simulink model "SimNL_Subsystems"  (R2016b)
settings: Solver=VariableStepAuto  StartTime=0.0  StopTime=10  FixedStep=SampleTime  RelTol=1e-3
values from neighbouring files (symbols this model uses):
  AC = []    [SetupNL.m]
undefined symbols (not defined in the file or in its folder): Env, Sim
libraries: OpenFlightUtilLib x17, SimCoreLib x3
(part 1 of 2)
settings Model: LastModifiedBy=rega0051
settings SolverCC: AlgebraicLoopSolver=LineSearch  AutoInsertRateTranBlk=on
settings DataIOCC: ExternalInput=simIn  FinalStateName=simStatesFinal  InitialState=simStatesInit  SaveOutput=off  SignalLogging=off  DSMLogging=off  StreamVariableName=simStream  SaveTime=off  StateSaveName=simStates  TimeSaveName=simTime  OutputSaveName=simOut  SignalLoggingName=simLog  DSMLoggingName=simData
settings OptimizationCC: ExpressionDepthLimit=2147483647  LifeSpan=inf
settings DebuggingCC: SignalInfNanChecking=warning  SaveWithParameterizedLinksMsg=none  UnderspecifiedInitializationDetection=Classic  MergeDetectMultiDrivingBlocksExec=none  CheckMatrixSingularityMsg=warning  UnnecessaryDatatypeConvMsg=warning  SignalLabelMismatchMsg=warning  SFcnCompatibilityMsg=warning  UniqueDataStoreMsg=error  ModelReferenceIOMsg=warning  ModelReferenceVersionMismatchMessage=warning  ModelReferenceIOMismatchMessage=warning  ModelReferenceExtraNoncontSigs=none  StateNameClashWarn=warning  StrictBusMsg=WarnOnBusTreatedAsVector  NonBusSignalsTreatedAsBus=warning  SFUnexpectedBacktrackingDiag=warning  SFNoUnconditionalDefaultTransitionDiag=warning  SFExecutionAtInitializationDiag=none
settings HardwareCC: ProdBitPerPointer=32  ProdBitPerSizeT=32  ProdBitPerPtrDiffT=32  ProdLargestAtomicFloat=None  ProdWordSize=32  ProdHWDeviceType=Custom Processor->Custom
settings ModelReferenceCC: ModelReferenceMinAlgLoopOccurrences=on
settings GRTTargetCC: TargetLangStandard=C89/C90 (ANSI)  GeneratePreprocessorConditionals=Disable all  CombineOutputUpdateFcns=off  GRTInterface=on
settings ConfigComp: CovMetricSettings=dw  CovHtmlReporting=on  CovSaveCumulativeToWorkspaceVar=on  CovSaveSingleToWorkspaceVar=on  CovExternalEMLEnable=off  CovSFcnEnable=off

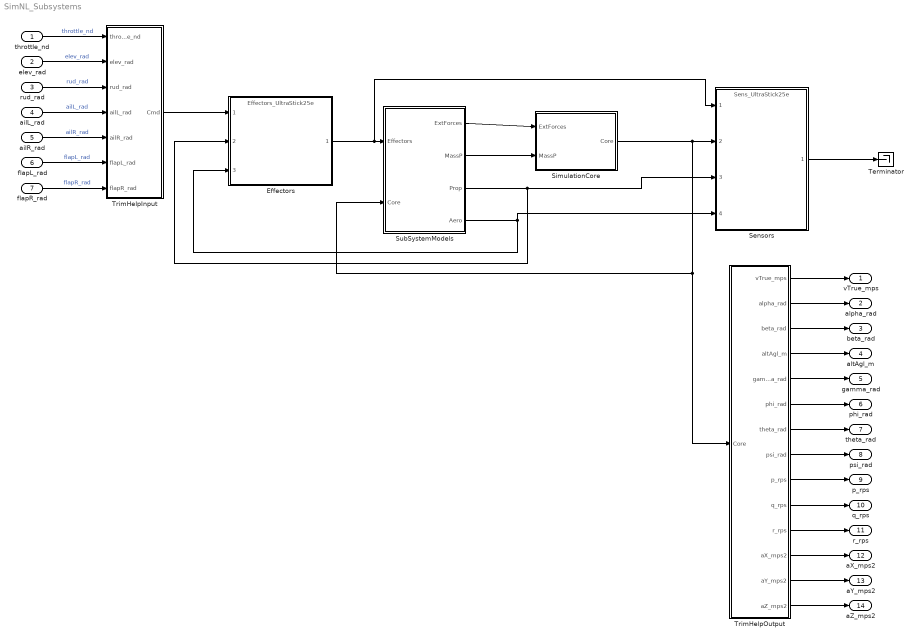
== system SimNL_Subsystems ==
  throttle_nd : Inport
  elev_rad : Inport  Port=2
  rud_rad : Inport  Port=3
  ailL_rad : Inport  Port=4
  ailR_rad : Inport  Port=5
  flapL_rad : Inport  Port=6
  flapR_rad : Inport  Port=7
  Effectors : ModelReference  ModelNameDialog=Effectors_UltraStick25e.slx  SimulationMode=Normal  ModelReferenceVersion=$Id: UAV_NL.mdl 1030 2014-05-21 20:23:20Z brtaylor $
  Sensors : ModelReference  ModelNameDialog=Sens_UltraStick25e.slx  SimulationMode=Normal  ModelReferenceVersion=1.78
  SimulationCore : Subsystem
  SubSystemModels : Subsystem
  Terminator : Terminator
  TrimHelpInput : Subsystem
  TrimHelpOutput : Subsystem
  vTrue_mps : Outport
  alpha_rad : Outport  Port=2
  beta_rad : Outport  Port=3
  altAgl_m : Outport  Port=4
  gamma_rad : Outport  Port=5
  phi_rad : Outport  Port=6
  theta_rad : Outport  Port=7
  psi_rad : Outport  Port=8
  p_rps : Outport  Port=9
  q_rps : Outport  Port=10
  r_rps : Outport  Port=11
  aX_mps2 : Outport  Port=12
  aY_mps2 : Outport  Port=13
  aZ_mps2 : Outport  Port=14
  wires:
  SimulationCore/1(Core) -> SubSystemModels/2(Core), TrimHelpOutput/1(Core), Sensors/2
  SubSystemModels/1(ExtForces) -> SimulationCore/1(ExtForces)
  SubSystemModels/2(MassP) -> SimulationCore/2(MassP)
  TrimHelpOutput/1(vTrue_mps) -> vTrue_mps/1
  TrimHelpOutput/2(alpha_rad) -> alpha_rad/1
  TrimHelpOutput/3(beta_rad) -> beta_rad/1
  TrimHelpOutput/4(altAgl_m) -> altAgl_m/1
  TrimHelpOutput/5(gamma_rad) -> gamma_rad/1
  TrimHelpOutput/6(phi_rad) -> phi_rad/1
  TrimHelpOutput/7(theta_rad) -> theta_rad/1
  TrimHelpOutput/8(psi_rad) -> psi_rad/1
  TrimHelpOutput/9(p_rps) -> p_rps/1
  TrimHelpOutput/10(q_rps) -> q_rps/1
  TrimHelpOutput/11(r_rps) -> r_rps/1
  TrimHelpOutput/12(aX_mps2) -> aX_mps2/1
  TrimHelpOutput/13(aY_mps2) -> aY_mps2/1
  TrimHelpOutput/14(aZ_mps2) -> aZ_mps2/1
  TrimHelpInput/1(Cmd) -> Effectors/1
  SubSystemModels/3(Prop) -> Sensors/3, Effectors/2
  flapR_rad/1 -> TrimHelpInput/7(flapR_rad)  "flapR_rad"
  flapL_rad/1 -> TrimHelpInput/6(flapL_rad)  "flapL_rad"
  ailR_rad/1 -> TrimHelpInput/5(ailR_rad)  "ailR_rad"
  ailL_rad/1 -> TrimHelpInput/4(ailL_rad)  "ailL_rad"
  rud_rad/1 -> TrimHelpInput/3(rud_rad)  "rud_rad"
  elev_rad/1 -> TrimHelpInput/2(elev_rad)  "elev_rad"
  throttle_nd/1 -> TrimHelpInput/1(throttle_nd)  "throttle_nd"
  Sensors/1 -> Terminator/1
  SubSystemModels/4(Aero) -> Effectors/3, Sensors/4
  Effectors/1 -> Sensors/1, SubSystemModels/1(Effectors)

== system SimNL_Subsystems/SimulationCore ==
  ExtForces : Inport
  MassP : Inport  Port=2
  AuxiliaryEquations : Subsystem
      settings: MinAlgLoopOccurrences=on
  Bus Creator : BusCreator  Inputs=3  OutDataTypeStr=Bus: BusCore
      settings: AttributesFormatString=%<OutDataTypeStr>  InheritFromInputs=off
  EnvModel : Subsystem
      settings: MinAlgLoopOccurrences=on
  Eom_VarLocalLevelQuat : Subsystem
  Core : Outport
  wires:
  EnvModel/1(Env) -> Eom_VarLocalLevelQuat/3(Env), AuxiliaryEquations/2(Env), Bus Creator/3
  Bus Creator/1 -> EnvModel/1(Core), Core/1  "BusCore"
  AuxiliaryEquations/1(Aux) -> Bus Creator/2
  Eom_VarLocalLevelQuat/1(Eom) -> Bus Creator/1, AuxiliaryEquations/1(Eom)
  ExtForces/1 -> Eom_VarLocalLevelQuat/1(ExtForces)
  MassP/1 -> Eom_VarLocalLevelQuat/2(MassP)

== system SimNL_Subsystems/SubSystemModels ==
  Effectors : Inport
  Core : Inport  Port=2
  Aero_VarGen : Subsystem
  MassProp_Const : Subsystem
  Prop_VarCoefPoly1 : Subsystem
  SumExternalForces : Subsystem
  ExtForces : Outport
  MassP : Outport  Port=2
  Prop : Outport  Port=3
  Aero : Outport  Port=4
  wires:
  MassProp_Const/1(MassP) -> MassP/1
  SumExternalForces/1(ExtForce) -> ExtForces/1
  Effectors/1 -> Prop_VarCoefPoly1/1(Effectors), Aero_VarGen/1(Effectors)
  Core/1 -> Prop_VarCoefPoly1/2(Core), Aero_VarGen/2(Core)
  Aero_VarGen/1(Aero) -> Aero/1, SumExternalForces/1(Aero)
  Prop_VarCoefPoly1/1(Prop) -> SumExternalForces/2(Prop), Prop/1

== system SimNL_Subsystems/TrimHelpInput ==
  throttle_nd : Inport
  elev_rad : Inport  Port=2
  rud_rad : Inport  Port=3
  ailL_rad : Inport  Port=4
  ailR_rad : Inport  Port=5
  flapL_rad : Inport  Port=6
  flapR_rad : Inport  Port=7
  Bus Creator3 : BusCreator  Inputs=7  OutDataTypeStr=Bus: BusCmd
      settings: AttributesFormatString=%<OutDataTypeStr>  InheritFromInputs=off
  Cmd : Outport  OutDataTypeStr=Bus: BusCmd  SampleTime=0
      settings: AttributesFormatString=%<OutDataTypeStr>
  wires:
  Bus Creator3/1 -> Cmd/1  "BusCmd"
  throttle_nd/1 -> Bus Creator3/1
  elev_rad/1 -> Bus Creator3/2
  ailL_rad/1 -> Bus Creator3/4
  rud_rad/1 -> Bus Creator3/3
  flapL_rad/1 -> Bus Creator3/6
  ailR_rad/1 -> Bus Creator3/5
  flapR_rad/1 -> Bus Creator3/7

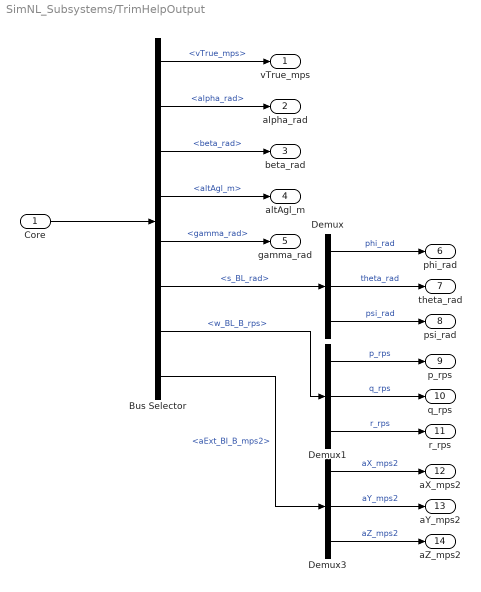
== system SimNL_Subsystems/TrimHelpOutput ==
  Core : Inport
  Bus Selector : BusSelector  OutputSignals=BusAux.BusFlow.vTrue_mps,BusAux.BusFlow.alpha_rad,BusAux.BusFlow.beta_rad,BusAux.BusNav.altAgl_m,BusAux.BusNav.gamma_rad,BusEom.s_BL_rad,BusEom.w_BL_B_rps,BusEom.aExt_BI_B_mps2
  Demux : Demux  Outputs=3
  Demux1 : Demux  Outputs=3
  Demux3 : Demux  Outputs=3
  vTrue_mps : Outport
  alpha_rad : Outport  Port=2
  beta_rad : Outport  Port=3
  altAgl_m : Outport  Port=4
  gamma_rad : Outport  Port=5
  phi_rad : Outport  Port=6
  theta_rad : Outport  Port=7
  psi_rad : Outport  Port=8
  p_rps : Outport  Port=9
  q_rps : Outport  Port=10
  r_rps : Outport  Port=11
  aX_mps2 : Outport  Port=12
  aY_mps2 : Outport  Port=13
  aZ_mps2 : Outport  Port=14
  wires:
  Core/1 -> Bus Selector/1
  Bus Selector/1 -> vTrue_mps/1  "<vTrue_mps>"
  Bus Selector/2 -> alpha_rad/1  "<alpha_rad>"
  Bus Selector/3 -> beta_rad/1  "<beta_rad>"
  Bus Selector/4 -> altAgl_m/1  "<altAgl_m>"
  Bus Selector/5 -> gamma_rad/1  "<gamma_rad>"
  Bus Selector/6 -> Demux/1  "<s_BL_rad>"
  Bus Selector/7 -> Demux1/1  "<w_BL_B_rps>"
  Demux/1 -> phi_rad/1  "phi_rad"
  Demux/2 -> theta_rad/1  "theta_rad"
  Demux/3 -> psi_rad/1  "psi_rad"
  Demux1/1 -> p_rps/1  "p_rps"
  Demux1/2 -> q_rps/1  "q_rps"
  Demux1/3 -> r_rps/1  "r_rps"
  Bus Selector/8 -> Demux3/1  "<aExt_BI_B_mps2>"
  Demux3/2 -> aY_mps2/1  "aY_mps2"
  Demux3/3 -> aZ_mps2/1  "aZ_mps2"
  Demux3/1 -> aX_mps2/1  "aX_mps2"

== system SimNL_Subsystems/SimulationCore/AuxiliaryEquations ==
  Eom : Inport  OutDataTypeStr=Bus: BusEom
  Env : Inport  Port=2  OutDataTypeStr=Bus: BusEnv
  Bus Creator2 : BusCreator  Inputs=2  OutDataTypeStr=Bus: BusAux
      settings: AttributesFormatString=%<OutDataTypeStr>  InheritFromInputs=off
  FlowConditions : SimCoreLib/FlowConditions
  NavEquations : SimCoreLib/NavEquations
  Aux : Outport
  wires:
  Eom/1 -> NavEquations/1, FlowConditions/1
  FlowConditions/1 -> Bus Creator2/1
  NavEquations/1 -> Bus Creator2/2
  Env/1 -> NavEquations/2, FlowConditions/2
  Bus Creator2/1 -> Aux/1  "BusAux"

== system SimNL_Subsystems/SimulationCore/EnvModel ==
  Core : Inport
  AtmosphereModel : Subsystem
  Bus Creator1 : BusCreator  Inputs=4  OutDataTypeStr=Bus: BusEnv
      settings: AttributesFormatString=%<OutDataTypeStr>
  GravityModel : Subsystem
  MagneticModel : Subsystem
  TerrainModel : Subsystem
  Env : Outport
  wires:
  Bus Creator1/1 -> Env/1  "BusEnv"
  Core/1 -> AtmosphereModel/1(Core), MagneticModel/1(Core), GravityModel/1(Core)
  AtmosphereModel/1(Atmos) -> Bus Creator1/1
  TerrainModel/1(Terr) -> Bus Creator1/2
  GravityModel/1(Grav) -> Bus Creator1/3
  MagneticModel/1(Mag) -> Bus Creator1/4

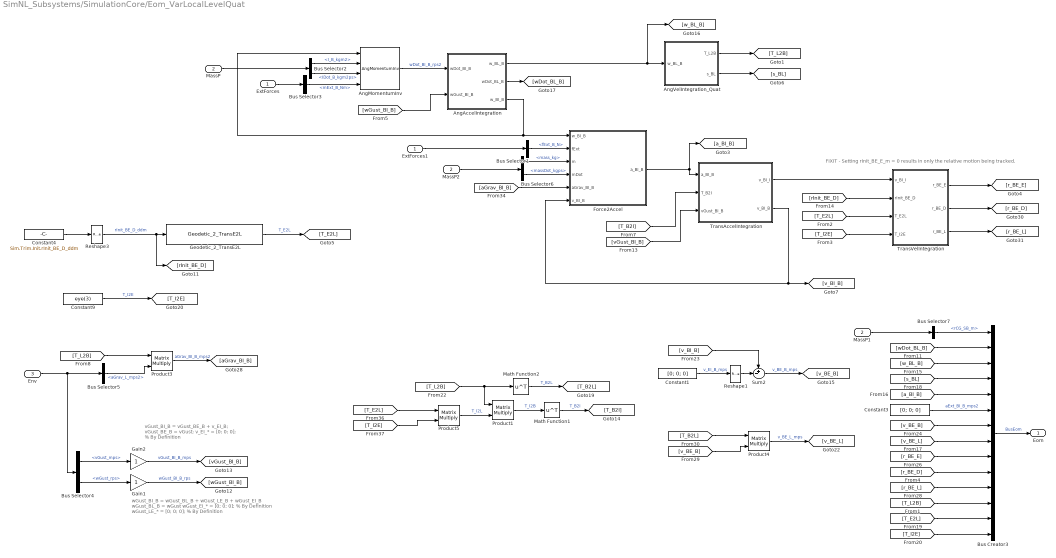
== system SimNL_Subsystems/SimulationCore/Eom_VarLocalLevelQuat ==
  note: FIXIT - Setting rInit_BE_E_m = 0 results in only the relative motion being tracked.
  note: vGust_BI_B = vGust_BE_B + v_EI_B;
      | vGust_BE_B = vGust;
      | v_EI_* = [0; 0; 0]; % By Definition
  note: wGust_BI_B = wGust_BL_B + wGust_LE_B + wGust_EI_B
      | wGust_BL_B = wGust
      | wGust_EI_* = [0; 0; 0]; % By Definition
      | wGust_LE_* = [0; 0; 0]; % By Definition
  ExtForces : Inport  OutDataTypeStr=Bus: BusExtForce
      settings: AttributesFormatString=%<OutDataTypeStr>
  MassP : Inport  Port=2  OutDataTypeStr=Bus: BusMassP
      settings: AttributesFormatString=%<OutDataTypeStr>
  Env : Inport  Port=3  OutDataTypeStr=Bus: BusEnv
      settings: AttributesFormatString=%<OutDataTypeStr>
  AngAccelIntegration : Subsystem
  AngMomentumInv : OpenFlightUtilLib/Kinematics and Dynamics/AngMomentumInv
  AngVelIntegration_Quat : Subsystem
  Bus Selector1 : BusSelector  OutputSignals=fExt_B_N
  Bus Selector2 : BusSelector  OutputSignals=I_B_kgm2,IDot_B_kgm2ps
  Bus Selector3 : BusSelector  OutputSignals=mExt_B_Nm
  Bus Selector4 : BusSelector  OutputSignals=BusAtmos.vGust_mps,BusAtmos.wGust_rps
  Bus Selector5 : BusSelector  OutputSignals=BusGrav.aGrav_L_mps2
  Bus Selector6 : BusSelector  OutputSignals=mass_kg,massDot_kgps
  Bus Selector7 : BusSelector  OutputSignals=rCG_SB_m
  Bus Creator3 : BusCreator  Inputs=14  OutDataTypeStr=Bus: BusEom
      settings: AttributesFormatString=%<OutDataTypeStr>  InheritFromInputs=off
  Constant1 : Constant  Value=[0; 0; 0]
      settings: AttributesFormatString=%<Value>
  Constant3 : Constant  Value=[0; 0; 0]
      settings: AttributesFormatString=%<Value>
  Constant4 : Constant  Value=Sim.Trim.Init.rInit_BE_D_ddm
      settings: AttributesFormatString=%<Value>
  Constant9 : Constant  Value=eye(3)
      settings: AttributesFormatString=%<Value>
  ExtForces1 : InportShadow  OutDataTypeStr=Bus: BusExtForce
      settings: AttributesFormatString=%<OutDataTypeStr>
  Force2Accel : Subsystem
  Gain1 : Gain
  Gain2 : Gain
  Geodetic_2_TransE2L : OpenFlightUtilLib/Transformations/Geodetic_2_TransE2L
  MassP1 : InportShadow  Port=2  OutDataTypeStr=Bus: BusMassP
      settings: AttributesFormatString=%<OutDataTypeStr>
  MassP2 : InportShadow  Port=2  OutDataTypeStr=Bus: BusMassP
      settings: AttributesFormatString=%<OutDataTypeStr>
  Math Function1 : Math  Operator=transpose  SaturateOnIntegerOverflow=on
  Math Function2 : Math  Operator=transpose  SaturateOnIntegerOverflow=on
  Product{1,3..5} (4 alike) : Product  Inputs=**  Multiplication=Matrix(*)  RndMeth=Zero
  Reshape1 : Reshape  OutputDimensionality=Column vector (2-D)  OutputDimensions=[3,1]
  Reshape3 : Reshape  OutputDimensionality=Column vector (2-D)  OutputDimensions=[3,1]
  Sum2 : Sum  Inputs=+-|
  TransAccelIntegration : Subsystem
  TransVelIntegration : Subsystem
  Eom : Outport  OutDataTypeStr=Bus: BusEom
      settings: AttributesFormatString=%<OutDataTypeStr>
  wires:
  Reshape3/1 -> Geodetic_2_TransE2L/1, [rInit_BE_D]  "rInit_BE_D_ddm"
  Math Function1/1 -> [T_B2I]  "T_B2I"
  Product1/1 -> Math Function1/1  "T_I2B"
  [T_B2I] -> TransAccelIntegration/2(T_B2I)
  TransVelIntegration/1(r_BE_E) -> [r_BE_E]
  TransAccelIntegration/1(v_BI_I) -> TransVelIntegration/1(v_BI_I)
  Bus Selector6/2 -> Force2Accel/4(mDot)  "<massDot_kgps>"
  Bus Selector6/1 -> Force2Accel/3(m)  "<mass_kg>"
  Product3/1 -> [aGrav_BI_B]  "aGrav_BI_B_mps2"
  AngVelIntegration_Quat/1(T_L2B) -> [T_L2B]
  Bus Selector1/1 -> Force2Accel/2(fExt)  "<fExt_B_N>"
  Bus Creator3/1 -> Eom/1  "BusEom"
  [T_L2B] -> Bus Creator3/12
  ExtForces1/1 -> Bus Selector1/1
  Bus Selector5/1 -> Product3/2  "<aGrav_L_mps2>"
  [T_L2B] -> Product3/1
  AngVelIntegration_Quat/2(s_BL) -> [s_BL]
  Force2Accel/1(a_BI_B) -> [a_BI_B], TransAccelIntegration/1(a_BI_B)
  AngMomentumInv/1 -> AngAccelIntegration/1(wDot_BI_B)  "wDot_BI_B_rps2"
  Bus Selector2/1 -> AngMomentumInv/2  "<I_B_kgm2>"
  Bus Selector2/2 -> AngMomentumInv/3  "<IDot_B_kgm2ps>"
  Bus Selector3/1 -> AngMomentumInv/4  "<mExt_B_Nm>"
  [s_BL] -> Bus Creator3/4
  [a_BI_B] -> Bus Creator3/5
  [r_BE_D] -> Bus Creator3/10
  [w_BL_B] -> Bus Creator3/3
  [wDot_BL_B] -> Bus Creator3/2
  [v_BE_L] -> Bus Creator3/8
  AngAccelIntegration/1(w_BL_B) -> [w_BL_B], AngVelIntegration_Quat/1(w_BL_B)
  [T_E2L] -> Bus Creator3/13
  [T_I2E] -> Bus Creator3/14
  Geodetic_2_TransE2L/1 -> [T_E2L]  "T_E2L"
  Constant9/1 -> [T_I2E]  "T_I2E"
  [T_L2B] -> Product1/1, Math Function2/1
  Product4/1 -> [v_BE_L]  "v_BE_L_mps"
  [r_BE_L] -> Bus Creator3/11
  [v_BE_B] -> Product4/2
  [T_B2L] -> Product4/1
  Product5/1 -> Product1/2  "T_I2L"
  Bus Selector4/1 -> Gain2/1  "<vGust_mps>"
  [aGrav_BI_B] -> Force2Accel/5(aGrav_BI_B)
  AngAccelIntegration/2(wDot_BL_B) -> [wDot_BL_B]
  TransVelIntegration/2(r_BE_D) -> [r_BE_D]
  TransVelIntegration/3(r_BE_L) -> [r_BE_L]
  [rInit_BE_D] -> TransVelIntegration/2(rInit_BE_D)
  [T_I2E] -> Product5/2
  [T_E2L] -> Product5/1
  MassP/1 -> Bus Selector2/1
  Bus Selector7/1 -> Bus Creator3/1  "<rCG_SB_m>"
  [wGust_BI_B] -> AngAccelIntegration/2(wGust_BI_B)
  Env/1 -> Bus Selector4/1, Bus Selector5/1
  Bus Selector4/2 -> Gain1/1  "<wGust_rps>"
  Gain2/1 -> [vGust_BI_B]  "vGust_BI_B_mps"
  Gain1/1 -> [wGust_BI_B]  "wGust_BI_B_rps"
  [vGust_BI_B] -> TransAccelIntegration/3(vGust_BI_B)
  [v_BE_B] -> Bus Creator3/7
  [r_BE_E] -> Bus Creator3/9
  [T_E2L] -> TransVelIntegration/3(T_E2L)
  Sum2/1 -> [v_BE_B]  "v_BE_B_mps"
  Constant1/1 -> Reshape1/1  "v_EI_B_mps"
  [v_BI_B] -> Sum2/1
  Math Function2/1 -> [T_B2L]  "T_B2L"
  Reshape1/1 -> Sum2/2
  AngAccelIntegration/3(w_BI_B) -> Force2Accel/1(w_BI_B), AngMomentumInv/1
  TransAccelIntegration/2(v_BI_B) -> [v_BI_B], Force2Accel/6(v_BI_B)
  Constant3/1 -> Bus Creator3/6  "aExt_BI_B_mps2"
  Constant4/1 -> Reshape3/1
  [T_I2E] -> TransVelIntegration/4(T_I2E)
  MassP1/1 -> Bus Selector7/1
  ExtForces/1 -> Bus Selector3/1
  MassP2/1 -> Bus Selector6/1

== system SimNL_Subsystems/SubSystemModels/Aero_VarGen ==
  note: Aero Force Coefficients are in the "Aero" reference frame [+downstream, +side, +Up(lift)] centered at the Aero Center
      | Aero Moment Coefficients are in the Body Frame, at the Aero Center
      |
      | Forces and Moments are output in the Body Frame
  Effectors : Inport  OutDataTypeStr=Bus: BusEff
      settings: AttributesFormatString=%<OutDataTypeStr>
  Core : Inport  Port=2  OutDataTypeStr=Bus: BusCore
      settings: AttributesFormatString=%<OutDataTypeStr>
  Aero2Body : Subsystem
  AeroCoefLookup : Subsystem
  Bus Creator1 : BusCreator  Inputs=2  OutDataTypeStr=Bus: BusAero
      settings: AttributesFormatString=%<OutDataTypeStr>  InheritFromInputs=off
  ComputeForces : Subsystem
  ComputeMoments : Subsystem
  Aero : Outport  OutDataTypeStr=Bus: BusAero
      settings: AttributesFormatString=%<OutDataTypeStr>
  wires:
  Effectors/1 -> AeroCoefLookup/1(Effectors)
  ComputeForces/1(Forces) -> Aero2Body/1(F_Aero)
  ComputeMoments/1(Moments) -> Aero2Body/2(M_B)
  Aero2Body/1(F_Body) -> Bus Creator1/1
  Aero2Body/2(M_Body) -> Bus Creator1/2
  AeroCoefLookup/1(CoefForces) -> ComputeForces/1(Force Coefficients)
  AeroCoefLookup/2(CoefMoments) -> ComputeMoments/1(Moment Coefficients)
  Bus Creator1/1 -> Aero/1  "BusAero"
  Core/1 -> ComputeForces/2(Core), ComputeMoments/2(Core), Aero2Body/3(Core), AeroCoefLookup/2(Core)

== system SimNL_Subsystems/SubSystemModels/MassProp_Const ==
  Bus Creator : BusCreator  Inputs=6  OutDataTypeStr=Bus: BusMassP
      settings: AttributesFormatString=%<OutDataTypeStr>  InheritFromInputs=off
  Constant1 : Constant  Value=AC.MassP.mass_kg
      settings: AttributesFormatString=%<Value>
  Constant2 : Constant  Value=AC.MassP.rCG_SB_m
      settings: AttributesFormatString=%<Value>
  Constant3 : Constant  Value=AC.MassP.I_B_kgm2
      settings: AttributesFormatString=%<Value>
  Constant4 : Constant  Value=0
      settings: AttributesFormatString=%<Value>
  Constant5 : Constant  Value=[0; 0; 0]
      settings: AttributesFormatString=%<Value>
  Constant6 : Constant  Value=zeros(3)
      settings: AttributesFormatString=%<Value>
  MassP : Outport
  wires:
  Bus Creator/1 -> MassP/1  "BusMassP"
  Constant1/1 -> Bus Creator/1  "mass_kg"
  Constant2/1 -> Bus Creator/3  "rCG_SB_m"
  Constant3/1 -> Bus Creator/5  "I_B_kgm2"
  Constant4/1 -> Bus Creator/2  "massDot_kgps"
  Constant5/1 -> Bus Creator/4  "rCG_B_m"
  Constant6/1 -> Bus Creator/6  "IDot_B_kgm2ps"

== system SimNL_Subsystems/SubSystemModels/Prop_VarCoefPoly1 ==
  Effectors : Inport  OutDataTypeStr=Bus: BusEff  SampleTime=0
      settings: AttributesFormatString=%<OutDataTypeStr>
  Core : Inport  Port=2  OutDataTypeStr=Bus: BusCore
      settings: AttributesFormatString=%<OutDataTypeStr>
  Bus Selector2 : BusSelector  OutputSignals=BusMotor.omega_rps
  Bus Selector3 : BusSelector  OutputSignals=BusMotor.torqueMotor_Nm
  Bus Creator1 : BusCreator  Inputs=5  OutDataTypeStr=Bus: BusProp
      settings: AttributesFormatString=%<OutDataTypeStr>  InheritFromInputs=off
  ComputeThrustTorque : Subsystem
  Core1 : InportShadow  Port=2  OutDataTypeStr=Bus: BusCore
      settings: AttributesFormatString=%<OutDataTypeStr>
  Gain8 : Gain  Gain=AC.Prop.spinDir_nd  SaturateOnIntegerOverflow=on  OutDataTypeStr=Inherit: Same as input  ParamDataTypeStr=Inherit: Same as input
      settings: AttributesFormatString=%<Gain>
  Prop2Body : Subsystem
  Prop : Outport  OutDataTypeStr=Bus: BusProp  SampleTime=0
      settings: AttributesFormatString=%<OutDataTypeStr>
  wires:
  Core/1 -> ComputeThrustTorque/2(Core)
  Prop2Body/2(M_Body) -> Bus Creator1/2
  ComputeThrustTorque/1(Thrust) -> Prop2Body/1(Thrust), Bus Creator1/4
  Prop2Body/1(F_Body) -> Bus Creator1/1
  Core1/1 -> Prop2Body/3(Core)
  Bus Creator1/1 -> Prop/1  "BusProp"
  Gain8/1 -> Prop2Body/2(Torque)
  Bus Selector2/1 -> Bus Creator1/3, ComputeThrustTorque/1(Omega)  "<omega_rps>"
  Effectors/1 -> Bus Selector3/1, Bus Selector2/1  "BusEff"
  Bus Selector3/1 -> Gain8/1  "<torqueMotor_Nm>"
  ComputeThrustTorque/2(Torque) -> Bus Creator1/5

== system SimNL_Subsystems/SubSystemModels/SumExternalForces ==
  Aero : Inport
  Prop : Inport  Port=2
  Bus Selector2 : BusSelector  OutputSignals=fProp_B_N,mProp_B_Nm
  Bus Selector3 : BusSelector  OutputSignals=fAero_B_N,mAero_B_Nm
  Bus Creator : BusCreator  Inputs=2  OutDataTypeStr=Bus: BusExtForce
      settings: AttributesFormatString=%<OutDataTypeStr>  InheritFromInputs=off
  Sum1 : Sum  Inputs=|++  SaturateOnIntegerOverflow=on
  Sum3 : Sum  Inputs=|++  SaturateOnIntegerOverflow=on
  ExtForce : Outport
  wires:
  Sum1/1 -> Bus Creator/2  "mExt_B_Nm"
  Sum3/1 -> Bus Creator/1  "fExt_B_N"
  Bus Creator/1 -> ExtForce/1  "BusExtForce"
  Prop/1 -> Bus Selector2/1
  Bus Selector2/1 -> Sum3/2  "<fProp_B_N>"
  Bus Selector2/2 -> Sum1/2  "<mProp_B_Nm>"
  Aero/1 -> Bus Selector3/1
  Bus Selector3/1 -> Sum3/1  "<fAero_B_N>"
  Bus Selector3/2 -> Sum1/1  "<mAero_B_Nm>"

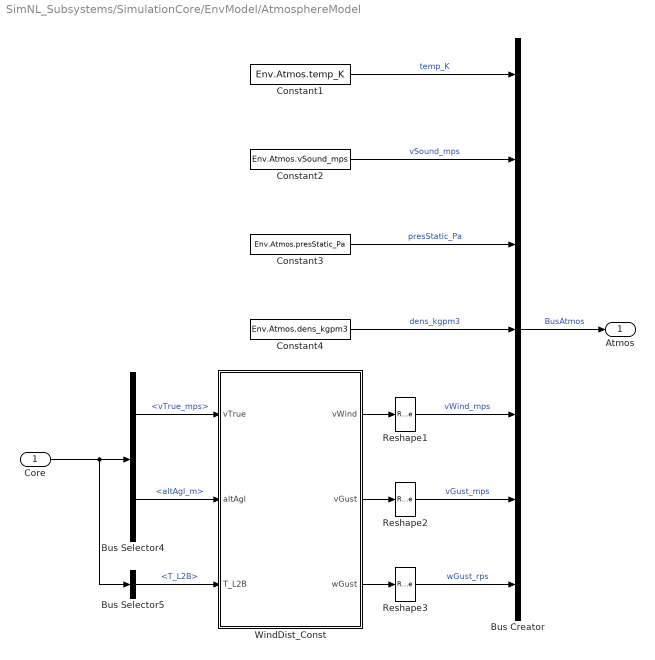
== system SimNL_Subsystems/SimulationCore/EnvModel/AtmosphereModel ==
  Core : Inport  OutDataTypeStr=Bus: BusCore
      settings: AttributesFormatString=%<OutDataTypeStr>
  Bus Creator : BusCreator  Inputs=7  OutDataTypeStr=Bus: BusAtmos
      settings: AttributesFormatString=%<OutDataTypeStr>
  Bus Selector4 : BusSelector  OutputSignals=BusAux.BusFlow.vTrue_mps,BusAux.BusNav.altAgl_m
  Bus Selector5 : BusSelector  OutputSignals=BusEom.T_L2B
  Constant1 : Constant  Value=Env.Atmos.temp_K
      settings: AttributesFormatString=%<Value>
  Constant2 : Constant  Value=Env.Atmos.vSound_mps
      settings: AttributesFormatString=%<Value>
  Constant3 : Constant  Value=Env.Atmos.presStatic_Pa
      settings: AttributesFormatString=%<Value>
  Constant4 : Constant  Value=Env.Atmos.dens_kgpm3
      settings: AttributesFormatString=%<Value>
  Reshape1 : Reshape  OutputDimensionality=Column vector (2-D)  OutputDimensions=[3,1]
  Reshape2 : Reshape  OutputDimensionality=Column vector (2-D)  OutputDimensions=[3,1]
  Reshape3 : Reshape  OutputDimensionality=Column vector (2-D)  OutputDimensions=[3,1]
  WindDist_Const : Subsystem
      settings: MinAlgLoopOccurrences=on
  Atmos : Outport  OutDataTypeStr=Bus: BusAtmos
      settings: AttributesFormatString=%<OutDataTypeStr>
  wires:
  Reshape3/1 -> Bus Creator/7  "wGust_rps"
  Reshape2/1 -> Bus Creator/6  "vGust_mps"
  Reshape1/1 -> Bus Creator/5  "vWind_mps"
  Bus Creator/1 -> Atmos/1  "BusAtmos"
  Core/1 -> Bus Selector5/1, Bus Selector4/1
  Constant1/1 -> Bus Creator/1  "temp_K"
  WindDist_Const/1(vWind) -> Reshape1/1
  WindDist_Const/3(wGust) -> Reshape3/1
  Constant2/1 -> Bus Creator/2  "vSound_mps"
  Constant3/1 -> Bus Creator/3  "presStatic_Pa"
  WindDist_Const/2(vGust) -> Reshape2/1
  Constant4/1 -> Bus Creator/4  "dens_kgpm3"
  Bus Selector4/1 -> WindDist_Const/1(vTrue)  "<vTrue_mps>"
  Bus Selector4/2 -> WindDist_Const/2(altAgl)  "<altAgl_m>"
  Bus Selector5/1 -> WindDist_Const/3(T_L2B)  "<T_L2B>"

== system SimNL_Subsystems/SimulationCore/EnvModel/GravityModel ==
  Core : Inport  OutDataTypeStr=Bus: BusCore
      settings: AttributesFormatString=%<OutDataTypeStr>
  Bus Creator : BusCreator  Inputs=1  OutDataTypeStr=Bus: BusGrav
      settings: AttributesFormatString=%<OutDataTypeStr>
  Constant : Constant  Value=Env.Grav.aGrav_L_mps2  SampleTime=-1
      settings: AttributesFormatString=%<Value>
  Reshape1 : Reshape  OutputDimensionality=Column vector (2-D)  OutputDimensions=[3,1]
  declination : Terminator
  Grav : Outport  OutDataTypeStr=Bus: BusGrav
      settings: AttributesFormatString=%<OutDataTypeStr>
  wires:
  Constant/1 -> Reshape1/1
  Bus Creator/1 -> Grav/1  "BusGrav"
  Core/1 -> declination/1
  Reshape1/1 -> Bus Creator/1  "aGrav_L_mps2"

== system SimNL_Subsystems/SimulationCore/EnvModel/MagneticModel ==
  Core : Inport  OutDataTypeStr=Bus: BusCore
      settings: AttributesFormatString=%<OutDataTypeStr>
  Bus Creator1 : BusCreator  Inputs=1  OutDataTypeStr=Bus: BusMag
      settings: AttributesFormatString=%<OutDataTypeStr>  InheritFromInputs=off
  Constant : Constant  Value=Env.Mag.h_L_nT
      settings: AttributesFormatString=%<Value>
  Reshape1 : Reshape  OutputDimensionality=Column vector (2-D)  OutputDimensions=[3,1]
  declination : Terminator
  Mag : Outport  OutDataTypeStr=Bus: BusMag
      settings: AttributesFormatString=%<OutDataTypeStr>
  wires:
  Reshape1/1 -> Bus Creator1/1  "h_L_nT"
  Core/1 -> declination/1
  Constant/1 -> Reshape1/1
  Bus Creator1/1 -> Mag/1  "BusMag"

== system SimNL_Subsystems/SimulationCore/EnvModel/TerrainModel ==
  Bus Creator1 : BusCreator  Inputs=1  OutDataTypeStr=Bus: BusTerr
      settings: AttributesFormatString=%<OutDataTypeStr>
  Constant : Constant  Value=Env.Terr.altGrd_m  SampleTime=-1
      settings: AttributesFormatString=%<Value>
  Terr : Outport  OutDataTypeStr=Bus: BusTerr
      settings: AttributesFormatString=%<OutDataTypeStr>
  wires:
  Bus Creator1/1 -> Terr/1  "BusTerr"
  Constant/1 -> Bus Creator1/1  "altGrnd_m"

== system SimNL_Subsystems/SimulationCore/Eom_VarLocalLevelQuat/AngAccelIntegration ==
  note: w_BL_B = w_BI_B - w_EI_B - w_LE_B
      | w_EI_* = [0; 0; 0]; % Non-rotating Earth
      | w_LE_* = [0; 0; 0]; % Flat Earth
  note: wDot_BL_B = wDot_BI_B - wDot_EI_B - wDot_LE_B
      | wDot_EI_* = [0; 0; 0]; % By Definition
      | wDot_LE_* = [0; 0; 0]; % Flat Earth
  wDot_BI_B : Inport
  wGust_BI_B : Inport  Port=2
  Constant4 : Constant  Value=Sim.Trim.Init.wState_BI_B_rps
      settings: AttributesFormatString=%<Value>
  Gain : Gain
  Gain1 : Gain
  Integrator : Integrator  InitialConditionSource=external  ContinuousStateAttributes='wState_BI_B_rps'
      settings: AttributesFormatString=State: %<ContinuousStateAttributes>
  Sum2 : Sum  Inputs=|++  SaturateOnIntegerOverflow=on
  w_BL_B : Outport
  wDot_BL_B : Outport  Port=2
  w_BI_B : Outport  Port=3
  wires:
  Constant4/1 -> Integrator/2  "wInit_BI_B_rps"
  wGust_BI_B/1 -> Sum2/2
  Gain/1 -> wDot_BL_B/1  "wDot_BL_B_rps2"
  Gain1/1 -> w_BL_B/1  "w_BL_B_rps"
  wDot_BI_B/1 -> Gain/1, Integrator/1
  Integrator/1 -> Sum2/1  "w_BI_B_rps"
  Sum2/1 -> w_BI_B/1, Gain1/1  "w_BI_B_rps"

== system SimNL_Subsystems/SimulationCore/Eom_VarLocalLevelQuat/AngVelIntegration_Quat ==
  w_BL_B : Inport
  Constant4 : Constant  Value=Sim.Trim.Init.quatState
      settings: AttributesFormatString=%<Value>
  NormL2 : OpenFlightUtilLib/Math/NormL2
  Product2 : Product  Inputs=*/  RndMeth=Zero
  Quat2DCM321 : OpenFlightUtilLib/Transformations/Quat2DCM
  Quat2Euler : OpenFlightUtilLib/Transformations/Quat2Euler
  QuatDeriv : OpenFlightUtilLib/Transformations/QuatDeriv
  QuatInt : OpenFlightUtilLib/Transformations/QuatInt
  T_L2B : Outport
  s_BL : Outport  Port=2
  wires:
  Quat2Euler/1 -> s_BL/1  "s_BL_rad"
  Quat2DCM321/1 -> T_L2B/1  "T_L2B"
  NormL2/1 -> Product2/2
  QuatDeriv/1 -> QuatInt/1  "quatDot_BL_nd"
  QuatInt/1 -> Product2/1, NormL2/1
  Product2/1 -> Quat2Euler/1, Quat2DCM321/1, QuatDeriv/1  "quat_BL_nd"
  Constant4/1 -> QuatInt/2  "quatInit_BL_nd"
  w_BL_B/1 -> QuatDeriv/2

== system SimNL_Subsystems/SimulationCore/Eom_VarLocalLevelQuat/Force2Accel ==
  w_BI_B : Inport
  fExt : Inport  Port=2
  m : Inport  Port=3
  mDot : Inport  Port=4
  aGrav_BI_B : Inport  Port=5
  v_BI_B : Inport  Port=6
  Product : Product
  Sum2 : Sum  Inputs=|++  SaturateOnIntegerOverflow=on
  TransMomentumInv : OpenFlightUtilLib/Kinematics and Dynamics/TransMomentumInv
  m1 : InportShadow  Port=3
  a_BI_B : Outport
  wires:
  Sum2/1 -> TransMomentumInv/3  "aTot_BI_B_mps2"
  Product/1 -> Sum2/2
  m1/1 -> Product/1
  fExt/1 -> Sum2/1
  v_BI_B/1 -> TransMomentumInv/1
  w_BI_B/1 -> TransMomentumInv/5
  mDot/1 -> TransMomentumInv/4
  m/1 -> TransMomentumInv/2
  aGrav_BI_B/1 -> Product/2
  TransMomentumInv/1 -> a_BI_B/1  "a_BI_B_mps2"

== system SimNL_Subsystems/SimulationCore/Eom_VarLocalLevelQuat/TransAccelIntegration ==
  a_BI_B : Inport
  T_B2I : Inport  Port=2
  vGust_BI_B : Inport  Port=3
  Constant4 : Constant  Value=Sim.Trim.Init.vState_BI_B_mps
      settings: AttributesFormatString=%<Value>
  Integrator : Integrator  InitialConditionSource=external  ContinuousStateAttributes='vState_BI_B_mps'
      settings: AttributesFormatString=State: %<ContinuousStateAttributes>
  Product1 : Product  Inputs=**  Multiplication=Matrix(*)  RndMeth=Zero
  Sum2 : Sum  Inputs=|++  SaturateOnIntegerOverflow=on
  v_BI_I : Outport
  v_BI_B : Outport  Port=2
  wires:
  Integrator/1 -> Sum2/1
  vGust_BI_B/1 -> Sum2/2
  Sum2/1 -> Product1/2, v_BI_B/1  "v_BI_B_mps"
  a_BI_B/1 -> Integrator/1
  T_B2I/1 -> Product1/1
  Product1/1 -> v_BI_I/1  "v_BI_I_mps"
  Constant4/1 -> Integrator/2  "vInit_BI_B_mps"

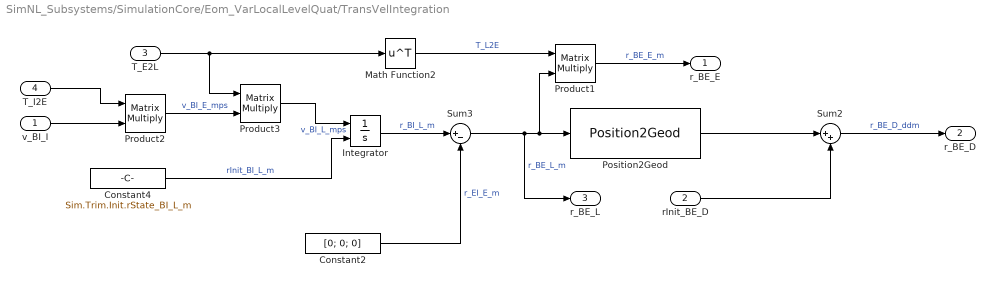
== system SimNL_Subsystems/SimulationCore/Eom_VarLocalLevelQuat/TransVelIntegration ==
  v_BI_I : Inport
  rInit_BE_D : Inport  Port=2
  T_E2L : Inport  Port=3
  T_I2E : Inport  Port=4
  Constant2 : Constant  Value=[0; 0; 0]
      settings: AttributesFormatString=%<Value>
  Constant4 : Constant  Value=Sim.Trim.Init.rState_BI_L_m
      settings: AttributesFormatString=%<Value>
  Integrator : Integrator  InitialConditionSource=external  ContinuousStateAttributes='rState_BI_L_m'
      settings: AttributesFormatString=State: %<ContinuousStateAttributes>
  Math Function2 : Math  Operator=transpose  SaturateOnIntegerOverflow=on
  Position2Geod : SimCoreLib/Position2Geod
  Product1 : Product  Inputs=**  Multiplication=Matrix(*)  RndMeth=Zero
  Product2 : Product  Inputs=**  Multiplication=Matrix(*)  RndMeth=Zero
  Product3 : Product  Inputs=**  Multiplication=Matrix(*)  RndMeth=Zero
  Sum2 : Sum  Inputs=|++
  Sum3 : Sum  Inputs=|+-
  r_BE_E : Outport
  r_BE_D : Outport  Port=2
  r_BE_L : Outport  Port=3
  wires:
  Product1/1 -> r_BE_E/1  "r_BE_E_m"
  Math Function2/1 -> Product1/1  "T_L2E"
  Product3/1 -> Integrator/1  "v_BI_L_mps"
  Product2/1 -> Product3/2  "v_BI_E_mps"
  T_I2E/1 -> Product2/1
  Constant4/1 -> Integrator/2  "rInit_BI_L_m"
  Constant2/1 -> Sum3/2  "r_EI_E_m"
  Sum3/1 -> Position2Geod/1, Product1/2, r_BE_L/1  "r_BE_L_m"
  rInit_BE_D/1 -> Sum2/2
  Sum2/1 -> r_BE_D/1  "r_BE_D_ddm"
  T_E2L/1 -> Product3/1, Math Function2/1
  Position2Geod/1 -> Sum2/1
  Integrator/1 -> Sum3/1  "r_BI_L_m"
  v_BI_I/1 -> Product2/2

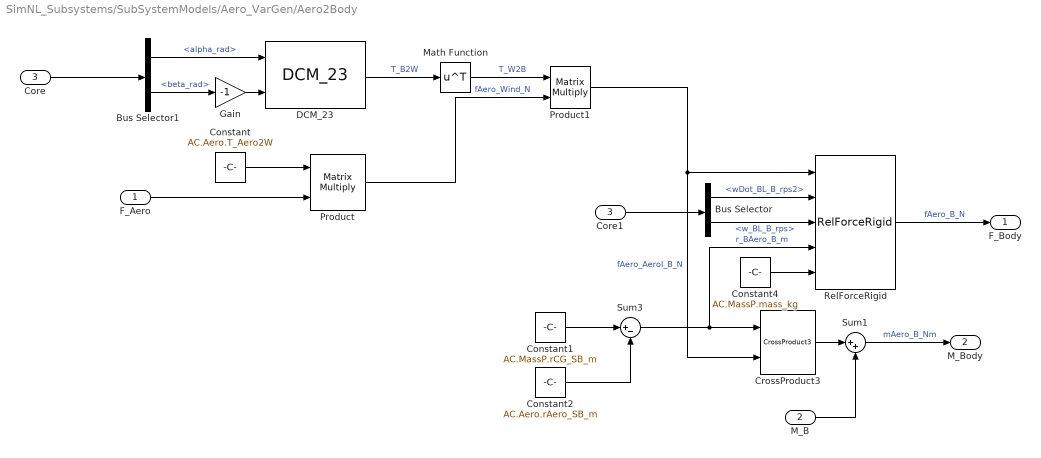
== system SimNL_Subsystems/SubSystemModels/Aero_VarGen/Aero2Body ==
  F_Aero : Inport
  M_B : Inport  Port=2
  Core : Inport  Port=3
  Bus Selector : BusSelector  OutputSignals=BusEom.wDot_BL_B_rps2,BusEom.w_BL_B_rps
  Bus Selector1 : BusSelector  OutputSignals=BusAux.BusFlow.alpha_rad,BusAux.BusFlow.beta_rad
  Constant : Constant  Value=AC.Aero.T_Aero2W
      settings: AttributesFormatString=%<Value>
  Constant1 : Constant  Value=AC.MassP.rCG_SB_m
      settings: AttributesFormatString=%<Value>
  Constant2 : Constant  Value=AC.Aero.rAero_SB_m
      settings: AttributesFormatString=%<Value>
  Constant4 : Constant  Value=AC.MassP.mass_kg
      settings: AttributesFormatString=%<Value>
  Core1 : InportShadow  Port=3
  CrossProduct3 : OpenFlightUtilLib/Math/CrossProduct3
  DCM_23 : OpenFlightUtilLib/Transformations/DCM_23
  Gain : Gain  Gain=-1
  Math Function : Math  Operator=transpose  SaturateOnIntegerOverflow=on
  Product : Product  Multiplication=Matrix(*)  RndMeth=Zero
  Product1 : Product  Multiplication=Matrix(*)  RndMeth=Zero
  RelForceRigid : OpenFlightUtilLib/Kinematics and Dynamics/RelForceRigid
  Sum1 : Sum  Inputs=|++  SaturateOnIntegerOverflow=on
  Sum3 : Sum  Inputs=|+-  SaturateOnIntegerOverflow=on
  F_Body : Outport
  M_Body : Outport  Port=2
  wires:
  Constant1/1 -> Sum3/1
  Constant2/1 -> Sum3/2
  Bus Selector/1 -> RelForceRigid/2  "<wDot_BL_B_rps2>"
  Bus Selector/2 -> RelForceRigid/3  "<w_BL_B_rps>"
  F_Aero/1 -> Product/2
  Constant/1 -> Product/1
  Core/1 -> Bus Selector1/1
  Math Function/1 -> Product1/1  "T_W2B"
  DCM_23/1 -> Math Function/1  "T_B2W"
  Product/1 -> Product1/2  "fAero_Wind_N"
  Product1/1 -> CrossProduct3/2, RelForceRigid/1  "fAero_AeroI_B_N"
  Sum3/1 -> RelForceRigid/4, CrossProduct3/1  "r_BAero_B_m"
  Core1/1 -> Bus Selector/1
  RelForceRigid/1 -> F_Body/1  "fAero_B_N"
  M_B/1 -> Sum1/2
  CrossProduct3/1 -> Sum1/1
  Sum1/1 -> M_Body/1  "mAero_B_Nm"
  Constant4/1 -> RelForceRigid/5
  Bus Selector1/1 -> DCM_23/1  "<alpha_rad>"
  Bus Selector1/2 -> Gain/1  "<beta_rad>"
  Gain/1 -> DCM_23/2

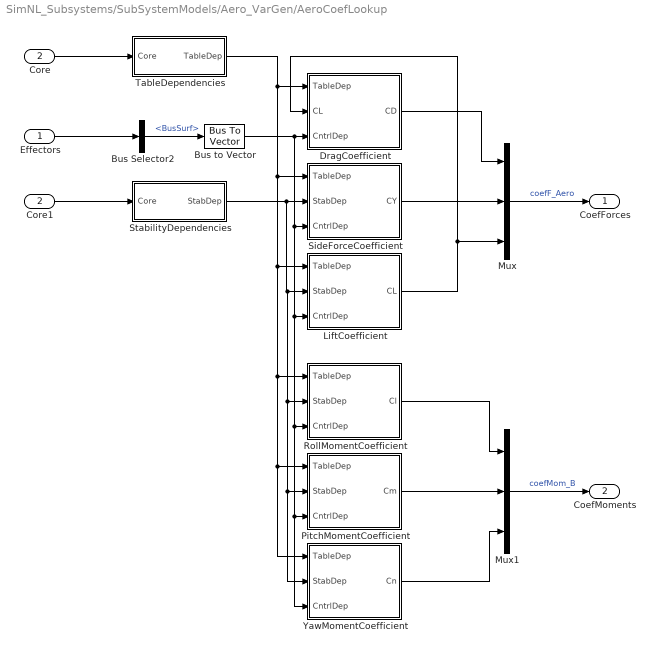
== system SimNL_Subsystems/SubSystemModels/Aero_VarGen/AeroCoefLookup ==
  Effectors : Inport
  Core : Inport  Port=2
  Bus Selector2 : BusSelector  OutputSignals=BusSurf
  Bus to Vector : BusToVector
  Core1 : InportShadow  Port=2
  DragCoefficient : Subsystem
  LiftCoefficient : Subsystem
  Mux : Mux  Inputs=3
  Mux1 : Mux  Inputs=3
  PitchMomentCoefficient : Subsystem
  RollMomentCoefficient : Subsystem
  SideForceCoefficient : Subsystem
  StabilityDependencies : Subsystem
  TableDependencies : Subsystem
  YawMomentCoefficient : Subsystem
  CoefForces : Outport
  CoefMoments : Outport  Port=2
  wires:
  Mux1/1 -> CoefMoments/1  "coefMom_B"
  SideForceCoefficient/1(CY) -> Mux/2
  PitchMomentCoefficient/1(Cm) -> Mux1/2
  Mux/1 -> CoefForces/1  "coefF_Aero"
  RollMomentCoefficient/1(Cl) -> Mux1/1
  LiftCoefficient/1(CL) -> DragCoefficient/2(CL), Mux/3
  YawMomentCoefficient/1(Cn) -> Mux1/3
  DragCoefficient/1(CD) -> Mux/1
  Bus Selector2/1 -> Bus to Vector/1  "<BusSurf>"
  TableDependencies/1(TableDep) -> SideForceCoefficient/1(TableDep), YawMomentCoefficient/1(TableDep), PitchMomentCoefficient/1(TableDep), RollMomentCoefficient/1(TableDep), LiftCoefficient/1(TableDep), DragCoefficient/1(TableDep)
  Effectors/1 -> Bus Selector2/1
  Core1/1 -> StabilityDependencies/1(Core)
  StabilityDependencies/1(StabDep) -> YawMomentCoefficient/2(StabDep), PitchMomentCoefficient/2(StabDep), RollMomentCoefficient/2(StabDep), LiftCoefficient/2(StabDep), SideForceCoefficient/2(StabDep)
  Bus to Vector/1 -> YawMomentCoefficient/3(CntrlDep), PitchMomentCoefficient/3(CntrlDep), RollMomentCoefficient/3(CntrlDep), LiftCoefficient/3(CntrlDep), SideForceCoefficient/3(CntrlDep), DragCoefficient/3(CntrlDep)
  Core/1 -> TableDependencies/1(Core)

== system SimNL_Subsystems/SubSystemModels/Aero_VarGen/ComputeForces ==
  Force Coefficients : Inport
  Core : Inport  Port=2
  Bus Selector : BusSelector  OutputSignals=BusAux.BusFlow.qBar_Pa
  Demux3 : Demux  Outputs=3
  Gain2 : Gain  Gain=AC.Aero.S  SaturateOnIntegerOverflow=on  OutDataTypeStr=Inherit: Same as input  ParamDataTypeStr=Inherit: Same as input
      settings: AttributesFormatString=%<Gain>
  Mux1 : Mux  Inputs=3
  Product6 : Product  SaturateOnIntegerOverflow=on  InputSameDT=on  OutDataTypeStr=Inherit: Same as first input
  Product7 : Product  SaturateOnIntegerOverflow=on  InputSameDT=on  OutDataTypeStr=Inherit: Same as first input
  Product8 : Product  SaturateOnIntegerOverflow=on  InputSameDT=on  OutDataTypeStr=Inherit: Same as first input
  Forces : Outport
  wires:
  Product6/1 -> Mux1/1  "fD_N"
  Product8/1 -> Mux1/3  "fL_N"
  Product7/1 -> Mux1/2  "fY_N"
  Mux1/1 -> Forces/1  "fAero_N"
  Demux3/2 -> Product7/1  "CY"
  Demux3/1 -> Product6/1  "CD"
  Demux3/3 -> Product8/1  "CL"
  Force Coefficients/1 -> Demux3/1
  Gain2/1 -> Product6/2, Product7/2, Product8/2
  Bus Selector/1 -> Gain2/1  "<qBar_Pa>"
  Core/1 -> Bus Selector/1

== system SimNL_Subsystems/SubSystemModels/Aero_VarGen/ComputeMoments ==
  Moment Coefficients : Inport
  Core : Inport  Port=2
  Bus Selector : BusSelector  OutputSignals=BusAux.BusFlow.qBar_Pa
  Demux3 : Demux  Outputs=3
  Gain1 : Gain  Gain=AC.Aero.b  SaturateOnIntegerOverflow=on  OutDataTypeStr=Inherit: Same as input  ParamDataTypeStr=Inherit: Same as input
      settings: AttributesFormatString=%<Gain>
  Gain2 : Gain  Gain=AC.Aero.S  SaturateOnIntegerOverflow=on  OutDataTypeStr=Inherit: Same as input  ParamDataTypeStr=Inherit: Same as input
      settings: AttributesFormatString=%<Gain>
  Gain3 : Gain  Gain=AC.Aero.b  SaturateOnIntegerOverflow=on  OutDataTypeStr=Inherit: Same as input  ParamDataTypeStr=Inherit: Same as input
      settings: AttributesFormatString=%<Gain>
  Gain4 : Gain  Gain=AC.Aero.c  SaturateOnIntegerOverflow=on  OutDataTypeStr=Inherit: Same as input  ParamDataTypeStr=Inherit: Same as input
      settings: AttributesFormatString=%<Gain>
  Mux1 : Mux  Inputs=3
  Product6 : Product  SaturateOnIntegerOverflow=on  InputSameDT=on  OutDataTypeStr=Inherit: Same as first input
  Product7 : Product  SaturateOnIntegerOverflow=on  InputSameDT=on  OutDataTypeStr=Inherit: Same as first input
  Product8 : Product  SaturateOnIntegerOverflow=on  InputSameDT=on  OutDataTypeStr=Inherit: Same as first input
  Moments : Outport
  wires:
  Product6/1 -> Mux1/1  "mL_Nm"
  Product8/1 -> Mux1/3  "mN_Nm"
  Moment Coefficients/1 -> Demux3/1
  Product7/1 -> Mux1/2  "mM_Nm"
  Gain3/1 -> Product8/2
  Mux1/1 -> Moments/1  "mAero_Nm"
  Gain1/1 -> Product6/2
  Gain2/1 -> Gain1/1, Gain4/1, Gain3/1
  Demux3/2 -> Product7/1  "Cm"
  Gain4/1 -> Product7/2
  Demux3/1 -> Product6/1  "Cl"
  Demux3/3 -> Product8/1  "Cn"
  Bus Selector/1 -> Gain2/1  "<qBar_Pa>"
  Core/1 -> Bus Selector/1

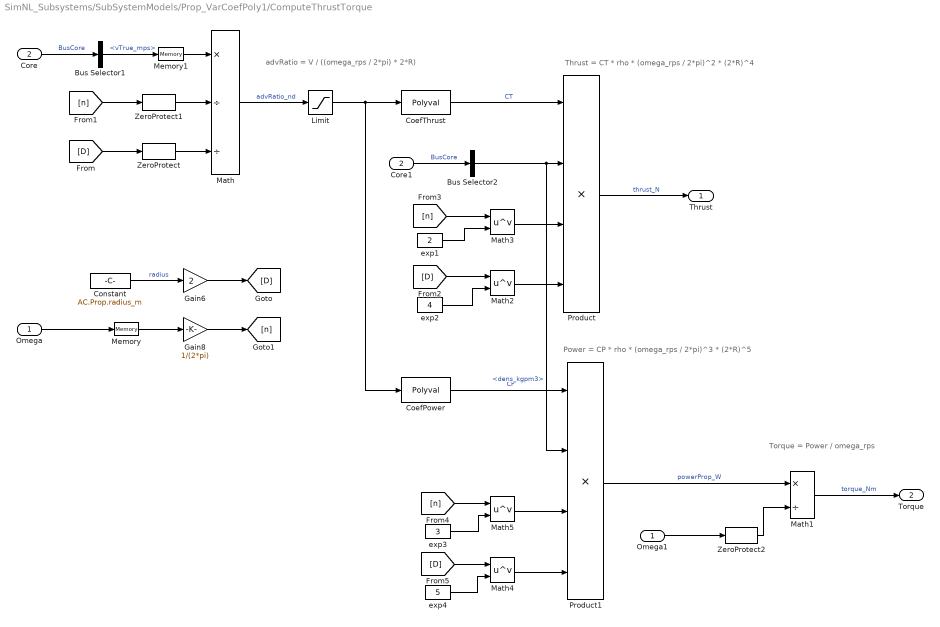
== system SimNL_Subsystems/SubSystemModels/Prop_VarCoefPoly1/ComputeThrustTorque ==
  note: Power = CP * rho * (omega_rps / 2*pi)^3 * (2*R)^5
  note: Thrust = CT * rho * (omega_rps / 2*pi)^2 * (2*R)^4
  note: advRatio = V / ((omega_rps / 2*pi) * 2*R)
  note: Torque = Power / omega_rps
  Omega : Inport  OutDataTypeStr=double
  Core : Inport  Port=2  OutDataTypeStr=double
  Bus Selector1 : BusSelector  OutputSignals=BusAux.BusFlow.vTrue_mps
  Bus Selector2 : BusSelector  OutputSignals=BusEnv.BusAtmos.dens_kgpm3
  CoefPower : Polyval  Coefs=AC.Prop.CP
      settings: AttributesFormatString=%<Coefs>
  CoefThrust : Polyval  Coefs=AC.Prop.CT
      settings: AttributesFormatString=%<Coefs>
  Constant : Constant  Value=AC.Prop.radius_m
      settings: AttributesFormatString=%<Value>
  Core1 : InportShadow  Port=2  OutDataTypeStr=double
  Gain6 : Gain  Gain=2  SaturateOnIntegerOverflow=on  OutDataTypeStr=Inherit: Same as input  ParamDataTypeStr=Inherit: Same as input
  Gain8 : Gain  Gain=1/(2*pi)  SaturateOnIntegerOverflow=on  OutDataTypeStr=Inherit: Same as input  ParamDataTypeStr=Inherit: Same as input
      settings: AttributesFormatString=%<Gain>
  Limit : Saturate  UpperLimit=0.7  LowerLimit=0
  Math : Product  Inputs=*//  SaturateOnIntegerOverflow=on  InputSameDT=on  OutDataTypeStr=Inherit: Same as first input
  Math1 : Product  Inputs=*/  SaturateOnIntegerOverflow=on  InputSameDT=on  OutDataTypeStr=Inherit: Same as first input
  Math{2..5} (4 alike) : Math  Operator=pow  SaturateOnIntegerOverflow=on
  Memory : Memory  X0=Sim.Trim.Init.omegaState_rps  InheritSampleTime=on  LinearizeMemory=on  StateIdentifier=omegaState_rps
      settings: AttributesFormatString=%<StateIdentifier>
  Memory1 : Memory  X0=Sim.Trim.Init.vTrueState_mps  InheritSampleTime=on  LinearizeMemory=on  StateIdentifier=vTrueState_mps
      settings: AttributesFormatString=%<StateIdentifier>
  Omega1 : InportShadow  OutDataTypeStr=double
  Product : Product  Inputs=4  SaturateOnIntegerOverflow=on  InputSameDT=on  OutDataTypeStr=Inherit: Same as first input
  Product1 : Product  Inputs=4  SaturateOnIntegerOverflow=on  InputSameDT=on  OutDataTypeStr=Inherit: Same as first input
  ZeroProtect : OpenFlightUtilLib/Math/ZeroProtect  epsilon=eps
  ZeroProtect1 : OpenFlightUtilLib/Math/ZeroProtect  epsilon=eps
  ZeroProtect2 : OpenFlightUtilLib/Math/ZeroProtect  epsilon=eps
  exp1 : Constant  Value=2
  exp2 : Constant  Value=4
  exp3 : Constant  Value=3
  exp4 : Constant  Value=5
  Thrust : Outport
  Torque : Outport  Port=2
  wires:
  Math1/1 -> Torque/1  "torque_Nm"
  ZeroProtect2/1 -> Math1/2
  Omega1/1 -> ZeroProtect2/1
  ZeroProtect1/1 -> Math/2
  ZeroProtect/1 -> Math/3
  [D] -> ZeroProtect/1
  [n] -> ZeroProtect1/1
  Gain8/1 -> [n]
  Omega/1 -> Memory/1
  Constant/1 -> Gain6/1  "radius"
  Gain6/1 -> [D]
  CoefPower/1 -> Product1/1  "CP"
  exp3/1 -> Math5/2
  [D] -> Math4/1
  [n] -> Math5/1
  Math5/1 -> Product1/3
  exp4/1 -> Math4/2
  Math4/1 -> Product1/4
  exp1/1 -> Math3/2
  [D] -> Math2/1
  [n] -> Math3/1
  Limit/1 -> CoefPower/1, CoefThrust/1
  Product1/1 -> Math1/1  "powerProp_W"
  Math/1 -> Limit/1  "advRatio_nd"
  Math3/1 -> Product/3
  exp2/1 -> Math2/2
  Math2/1 -> Product/4
  Product/1 -> Thrust/1  "thrust_N"
  CoefThrust/1 -> Product/1  "CT"
  Core/1 -> Bus Selector1/1  "BusCore"
  Bus Selector1/1 -> Memory1/1  "<vTrue_mps>"
  Bus Selector2/1 -> Product1/2, Product/2  "<dens_kgpm3>"
  Core1/1 -> Bus Selector2/1  "BusCore"
  Memory/1 -> Gain8/1
  Memory1/1 -> Math/1

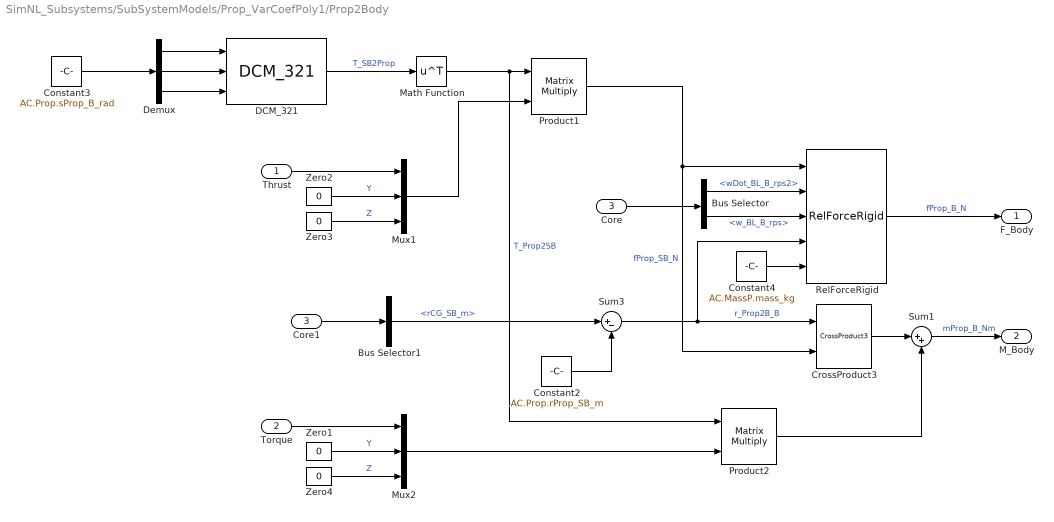
== system SimNL_Subsystems/SubSystemModels/Prop_VarCoefPoly1/Prop2Body ==
  Thrust : Inport
  Torque : Inport  Port=2
  Core : Inport  Port=3
  Bus Selector : BusSelector  OutputSignals=BusEom.wDot_BL_B_rps2,BusEom.w_BL_B_rps
  Bus Selector1 : BusSelector  OutputSignals=BusEom.rCG_SB_m
  Constant2 : Constant  Value=AC.Prop.rProp_SB_m
      settings: AttributesFormatString=%<Value>
  Constant3 : Constant  Value=AC.Prop.sProp_B_rad
      settings: AttributesFormatString=%<Value>
  Constant4 : Constant  Value=AC.MassP.mass_kg
      settings: AttributesFormatString=%<Value>
  Core1 : InportShadow  Port=3
  CrossProduct3 : OpenFlightUtilLib/Math/CrossProduct3
  DCM_321 : OpenFlightUtilLib/Transformations/DCM_321
  Demux : Demux  Outputs=3
  Math Function : Math  Operator=transpose  SaturateOnIntegerOverflow=on
  Mux1 : Mux  Inputs=3
  Mux2 : Mux  Inputs=3
  Product1 : Product  Multiplication=Matrix(*)  RndMeth=Zero
  Product2 : Product  Multiplication=Matrix(*)  RndMeth=Zero
  RelForceRigid : OpenFlightUtilLib/Kinematics and Dynamics/RelForceRigid
  Sum1 : Sum  Inputs=|++  SaturateOnIntegerOverflow=on
  Sum3 : Sum  Inputs=|+-  SaturateOnIntegerOverflow=on
  Zero{1..4} (4 alike) : Constant  Value=0
  F_Body : Outport
  M_Body : Outport  Port=2
  wires:
  Core1/1 -> Bus Selector1/1
  Mux2/1 -> Product2/2
  Torque/1 -> Mux2/1
  Zero1/1 -> Mux2/2  "Y"
  Zero4/1 -> Mux2/3  "Z"
  Mux1/1 -> Product1/2
  Zero2/1 -> Mux1/2  "Y"
  Zero3/1 -> Mux1/3  "Z"
  Constant4/1 -> RelForceRigid/5
  Product2/1 -> Sum1/2
  DCM_321/1 -> Math Function/1  "T_SB2Prop"
  Demux/2 -> DCM_321/2
  Demux/1 -> DCM_321/1
  Demux/3 -> DCM_321/3
  Constant3/1 -> Demux/1
  Sum1/1 -> M_Body/1  "mProp_B_Nm"
  CrossProduct3/1 -> Sum1/1
  RelForceRigid/1 -> F_Body/1  "fProp_B_N"
  Core/1 -> Bus Selector/1
  Sum3/1 -> RelForceRigid/4, CrossProduct3/1  "r_Prop2B_B"
  Product1/1 -> CrossProduct3/2, RelForceRigid/1  "fProp_SB_N"
  Math Function/1 -> Product1/1, Product2/1  "T_Prop2SB"
  Thrust/1 -> Mux1/1
  Bus Selector/2 -> RelForceRigid/3  "<w_BL_B_rps>"
  Bus Selector/1 -> RelForceRigid/2  "<wDot_BL_B_rps2>"
  Constant2/1 -> Sum3/2
  Bus Selector1/1 -> Sum3/1  "<rCG_SB_m>"

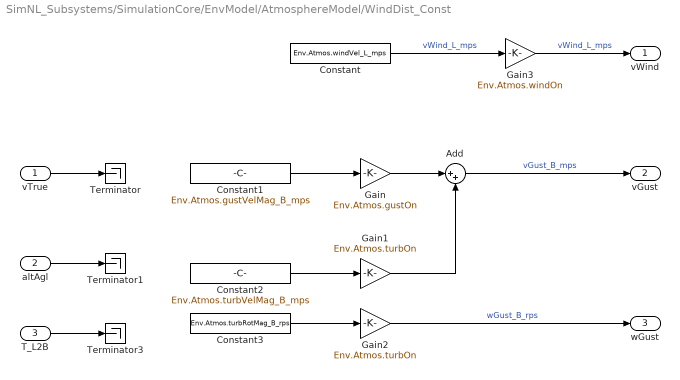
== system SimNL_Subsystems/SimulationCore/EnvModel/AtmosphereModel/WindDist_Const ==
  vTrue : Inport
  altAgl : Inport  Port=2
  T_L2B : Inport  Port=3
  Add : Sum  Inputs=|++
  Constant : Constant  Value=Env.Atmos.windVel_L_mps
      settings: AttributesFormatString=%<Value>
  Constant1 : Constant  Value=Env.Atmos.gustVelMag_B_mps
      settings: AttributesFormatString=%<Value>
  Constant2 : Constant  Value=Env.Atmos.turbVelMag_B_mps
      settings: AttributesFormatString=%<Value>
  Constant3 : Constant  Value=Env.Atmos.turbRotMag_B_rps
      settings: AttributesFormatString=%<Value>
  Gain : Gain  Gain=Env.Atmos.gustOn
      settings: AttributesFormatString=%<Gain>
  Gain1 : Gain  Gain=Env.Atmos.turbOn
      settings: AttributesFormatString=%<Gain>
  Gain2 : Gain  Gain=Env.Atmos.turbOn
      settings: AttributesFormatString=%<Gain>
  Gain3 : Gain  Gain=Env.Atmos.windOn
      settings: AttributesFormatString=%<Gain>
  Terminator : Terminator
  Terminator1 : Terminator
  Terminator3 : Terminator
  vWind : Outport
  vGust : Outport  Port=2
  wGust : Outport  Port=3
  wires:
  Gain2/1 -> wGust/1  "wGust_B_rps"
  Add/1 -> vGust/1  "vGust_B_mps"
  altAgl/1 -> Terminator1/1
  T_L2B/1 -> Terminator3/1
  Constant3/1 -> Gain2/1
  Gain1/1 -> Add/2
  Gain/1 -> Add/1
  Gain3/1 -> vWind/1  "vWind_L_mps"
  Constant2/1 -> Gain1/1
  Constant1/1 -> Gain/1
  Constant/1 -> Gain3/1  "vWind_L_mps"
  vTrue/1 -> Terminator/1

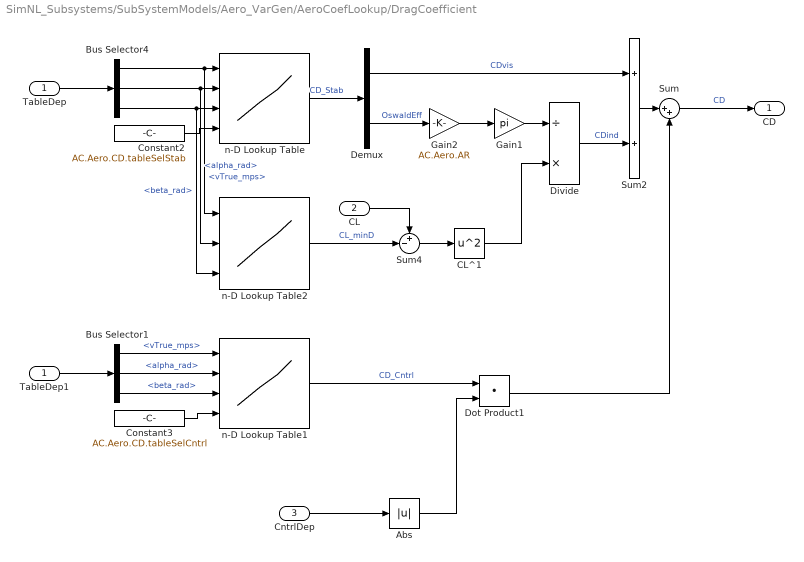
== system SimNL_Subsystems/SubSystemModels/Aero_VarGen/AeroCoefLookup/DragCoefficient ==
  TableDep : Inport
  CL : Inport  Port=2
  CntrlDep : Inport  Port=3
  Abs : Abs
  Bus Selector1 : BusSelector  OutputSignals=vTrue_mps,alpha_rad,beta_rad
  Bus Selector4 : BusSelector  OutputSignals=vTrue_mps,alpha_rad,beta_rad
  CL^1 : Math  Operator=square  SaturateOnIntegerOverflow=on
  Constant2 : Constant  Value=AC.Aero.CD.tableSelStab
      settings: AttributesFormatString=%<Value>
  Constant3 : Constant  Value=AC.Aero.CD.tableSelCntrl
      settings: AttributesFormatString=%<Value>
  Demux : Demux  Outputs=length(AC.Aero.CD.tableSelStab)
  Divide : Product  Inputs=/*
  Dot Product1 : DotProduct  InputSameDT=on  OutDataTypeStr=Inherit: Inherit via internal rule
  Gain1 : Gain  Gain=pi  SaturateOnIntegerOverflow=on  OutDataTypeStr=Inherit: Same as input  ParamDataTypeStr=Inherit: Same as input
      settings: AttributesFormatString=%<Gain>
  Gain2 : Gain  Gain=AC.Aero.AR  SaturateOnIntegerOverflow=on  OutDataTypeStr=Inherit: Same as input  ParamDataTypeStr=Inherit: Same as input
      settings: AttributesFormatString=%<Gain>
  Sum : Sum  Inputs=|++
  Sum2 : Sum  SaturateOnIntegerOverflow=on  InputSameDT=on  OutDataTypeStr=Inherit: Same as first input
  Sum4 : Sum  Inputs=+-|  SaturateOnIntegerOverflow=on  InputSameDT=on  OutDataTypeStr=Inherit: Same as first input
  TableDep1 : InportShadow
  n-D Lookup Table : Lookup_n-D  NumberOfTableDimensions=AC.Aero.tableDim  BreakpointsForDimension1=AC.Aero.breakPts{1}  BreakpointsForDimension2=AC.Aero.breakPts{2}  BreakpointsForDimension3=AC.Aero.breakPts{3}  BreakpointsForDimension4=AC.Aero.CD.tableSelStab  Table=AC.Aero.CD.tableStab  InternalRulePriority=Speed  RndMeth=Simplest  InputSameDT=on
      settings: AttributesFormatString=%<Table>
  n-D Lookup Table1 : Lookup_n-D  NumberOfTableDimensions=AC.Aero.tableDim  BreakpointsForDimension1=AC.Aero.breakPts{1}  BreakpointsForDimension2=AC.Aero.breakPts{2}  BreakpointsForDimension3=AC.Aero.breakPts{3}  BreakpointsForDimension4=AC.Aero.CD.tableSelCntrl  Table=AC.Aero.CD.tableCntrl  InternalRulePriority=Speed  RndMeth=Simplest  InputSameDT=on
      settings: AttributesFormatString=%<Table>
  n-D Lookup Table2 : Lookup_n-D  NumberOfTableDimensions=AC.Aero.tableDim - 1  BreakpointsForDimension1=AC.Aero.breakPts{1}  BreakpointsForDimension2=AC.Aero.breakPts{2}  BreakpointsForDimension3=AC.Aero.breakPts{3}  Table=AC.Aero.CL.minD  InternalRulePriority=Speed  RndMeth=Simplest  InputSameDT=on
      settings: AttributesFormatString=%<Table>
  CD : Outport
  wires:
  Sum/1 -> CD/1  "CD"
  Sum4/1 -> CL^1/1
  Bus Selector4/2 -> n-D Lookup Table2/2, n-D Lookup Table/2  "<alpha_rad>"
  Constant2/1 -> n-D Lookup Table/4
  Bus Selector4/1 -> n-D Lookup Table2/1, n-D Lookup Table/1  "<vTrue_mps>"
  n-D Lookup Table/1 -> Demux/1  "CD_Stab"
  Constant3/1 -> n-D Lookup Table1/4
  CntrlDep/1 -> Abs/1
  n-D Lookup Table1/1 -> Dot Product1/1  "CD_Cntrl"
  Dot Product1/1 -> Sum/2
  Demux/1 -> Sum2/1  "CDvis"
  Demux/2 -> Gain2/1  "OswaldEff"
  CL/1 -> Sum4/1
  n-D Lookup Table2/1 -> Sum4/2  "CL_minD"
  Gain2/1 -> Gain1/1
  CL^1/1 -> Divide/2
  Gain1/1 -> Divide/1
  Sum2/1 -> Sum/1
  Divide/1 -> Sum2/2  "CDind"
  Abs/1 -> Dot Product1/2
  Bus Selector4/3 -> n-D Lookup Table2/3, n-D Lookup Table/3  "<beta_rad>"
  Bus Selector1/1 -> n-D Lookup Table1/1  "<vTrue_mps>"
  Bus Selector1/3 -> n-D Lookup Table1/3  "<beta_rad>"
  Bus Selector1/2 -> n-D Lookup Table1/2  "<alpha_rad>"
  TableDep/1 -> Bus Selector4/1
  TableDep1/1 -> Bus Selector1/1

== system SimNL_Subsystems/SubSystemModels/Aero_VarGen/AeroCoefLookup/LiftCoefficient ==
  TableDep : Inport
  StabDep : Inport  Port=2
  CntrlDep : Inport  Port=3
  Bus Selector1 : BusSelector  OutputSignals=vTrue_mps,alpha_rad,beta_rad
  Bus Selector4 : BusSelector  OutputSignals=vTrue_mps,alpha_rad,beta_rad
  Constant1 : Constant  Value=AC.Aero.CL.tableSelCntrl
      settings: AttributesFormatString=%<Value>
  Constant2 : Constant  Value=AC.Aero.CL.tableSelStab
      settings: AttributesFormatString=%<Value>
  Dot Product : DotProduct  InputSameDT=on  OutDataTypeStr=Inherit: Inherit via internal rule
  Dot Product1 : DotProduct  InputSameDT=on  OutDataTypeStr=Inherit: Inherit via internal rule
  Sum : Sum  Inputs=|++
  n-D Lookup Table : Lookup_n-D  NumberOfTableDimensions=AC.Aero.tableDim  BreakpointsForDimension1=AC.Aero.breakPts{1}  BreakpointsForDimension2=AC.Aero.breakPts{2}  BreakpointsForDimension3=AC.Aero.breakPts{3}  BreakpointsForDimension4=AC.Aero.CL.tableSelStab  Table=AC.Aero.CL.tableStab  InternalRulePriority=Speed  RndMeth=Simplest  InputSameDT=on
      settings: AttributesFormatString=%<Table>
  n-D Lookup Table1 : Lookup_n-D  NumberOfTableDimensions=AC.Aero.tableDim  BreakpointsForDimension1=AC.Aero.breakPts{1}  BreakpointsForDimension2=AC.Aero.breakPts{2}  BreakpointsForDimension3=AC.Aero.breakPts{3}  BreakpointsForDimension4=AC.Aero.CL.tableSelCntrl  Table=AC.Aero.CL.tableCntrl  InternalRulePriority=Speed  RndMeth=Simplest  InputSameDT=on
      settings: AttributesFormatString=%<Table>
  CL : Outport
  wires:
  Dot Product/1 -> Sum/1
  Constant2/1 -> n-D Lookup Table/4
  n-D Lookup Table/1 -> Dot Product/1  "CL_Stab"
  StabDep/1 -> Dot Product/2
  TableDep/1 -> Bus Selector1/1, Bus Selector4/1
  Constant1/1 -> n-D Lookup Table1/4
  CntrlDep/1 -> Dot Product1/2
  n-D Lookup Table1/1 -> Dot Product1/1  "CL_Cntrl"
  Dot Product1/1 -> Sum/2
  Sum/1 -> CL/1  "CL"
  Bus Selector4/3 -> n-D Lookup Table/3  "<beta_rad>"
  Bus Selector4/2 -> n-D Lookup Table/2  "<alpha_rad>"
  Bus Selector4/1 -> n-D Lookup Table/1  "<vTrue_mps>"
  Bus Selector1/1 -> n-D Lookup Table1/1  "<vTrue_mps>"
  Bus Selector1/2 -> n-D Lookup Table1/2  "<alpha_rad>"
  Bus Selector1/3 -> n-D Lookup Table1/3  "<beta_rad>"
